simulink model "benchlink"  (R2024b)
settings: Solver=FixedStepDiscrete  StartTime=0.0  StopTime=0.005*16  RelTol=1e-3
model workspace (MAT data in the model file):
  socvcb = containers.Map
  socvcb.serialization.keys = {}
  socvcb.serialization.values = {}
  socvcb.serialization.uniformity = 0
  socvcb.serialization.keyType = 'double'
  socvcb.serialization.valueType = 'any'
values from neighbouring files (symbols this model uses):
  access = [32 0 4 36 32 0 4 36 32 0 4 36 ... (16 elements, 16x1)]    [all_variables.mat]
  qam_params =     [all_variables.mat]
undefined symbols (not defined in the file or in its folder): Add, j, QAM, rms, Shift
libraries: hdlsllib x53, simulink_need_slupdate x22, simulink x18, dspsigops x16, commdigbbndam3 x6, dsphdlmathfun2 x2, commchan3 x1, commrflib2 x1, dsphdlsigops2 x1, dspstat3 x1, dsphdlfiltering2 x1, simulink_extras x1
(part 1 of 5)
settings Model: ModifiedByFormat=The MathWorks Inc.  VariantFading=off  Creator=The MathWorks, Inc.  LastModifiedBy=The MathWorks Inc.
settings SolverCC: AlgebraicLoopSolver=TrustRegion  PositivePriorityOrder=on
settings DataIOCC: LimitDataPoints=on  SaveFormat=Array  SaveOutput=off  SaveTime=off  ReturnWorkspaceOutputs=off
settings OptimizationCC: BlockReduction=off  ConditionallyExecuteInputs=off  DefaultParameterBehavior=Inlined  EnhancedBackFolding=on  PassReuseOutputArgsAs=Individual arguments  MaxStackSize=64  OptimizeBlockOrder=speed  DifferentSizesBufferReuse=on  OptimizationCustomize=off  EfficientTunableParamExpr=on
settings DebuggingCC: AlgebraicLoopMsg=error  UnderspecifiedInitializationDetection=Classic  MergeDetectMultiDrivingBlocksExec=none  SolverPrmCheckMsg=warning  MultiTaskDSMMsg=warning  MultiTaskCondExecSysMsg=none  SingleTaskRateTransMsg=error  IntegerOverflowMsg=none  ParameterPrecisionLossMsg=none  ParameterTunabilityLossMsg=error  UnconnectedInputMsg=warning  UnconnectedOutputMsg=warning  UnconnectedLineMsg=warning  AllowSymbolicDim=off  StateNameClashWarn=warning  SFUnexpectedBacktrackingDiag=warning  SFNoUnconditionalDefaultTransitionDiag=warning  SFExecutionAtInitializationDiag=none  IntegerSaturationMsg=none  ArithmeticOperatorsInVariantConditions=warning
settings HardwareCC: ProdBitPerPointer=32  ProdBitPerSizeT=32  ProdBitPerPtrDiffT=32  ProdLargestAtomicFloat=None  ProdIntDivRoundTo=Undefined  ProdEndianess=Unspecified  ProdWordSize=32  ProdHWDeviceType=ASIC/FPGA->ASIC/FPGA  TargetBitPerLong=64  TargetBitPerPointer=64  TargetBitPerSizeT=64  TargetBitPerPtrDiffT=64  TargetLongLongMode=on  TargetIntDivRoundTo=Zero  TargetEndianess=LittleEndian  TargetWordSize=64  TargetHWDeviceType=Custom Processor->MATLAB Host Computer  ProdEqTarget=off
settings ModelReferenceCC: EnableRefExpFcnMdlSchedulingChecks=on  PropagateSignalLabelsOutOfModel=off
settings SFSimCC: SimUseLocalCustomCode=off  MATLABDynamicMemAlloc=off  CustomCodeUndefinedFunction=UseInterfaceOnly
settings RTWCC: Description=Embedded Coder  SystemTargetFile=ert.tlc  TemplateMakefile=ert_default_tmf  GenerateReport=on  RTWUseLocalCustomCode=off  Toolchain=Linaro AArch64 Linux v6.3.1  IncludeHyperlinkInReport=on  LaunchReport=on  GenerateTraceInfo=on  GenerateTraceReport=on  GenerateTraceReportSl=on  GenerateTraceReportSf=on  GenerateTraceReportEml=on  GPUComputeCapability=3.5  DLArmComputeVersion=19.05
settings CodeAppCC: ForceParamTrailComments=on  IgnoreCustomStorageClasses=off  OperatorAnnotations=on  SimulinkDataObjDesc=on  SFDataObjDesc=on  InsertBlockDesc=on
settings ERTTargetCC: InlinedParameterPlacement=Hierarchical  ERTCustomFileTemplate=example_file_process.tlc  DynamicArrayContainerType=coder::array
settings ConfigComp: CovMetricSettings=dw  CovSaveCumulativeToWorkspaceVar=on  CovSaveSingleToWorkspaceVar=on  CovExternalEMLEnable=off  CovSFcnEnable=off

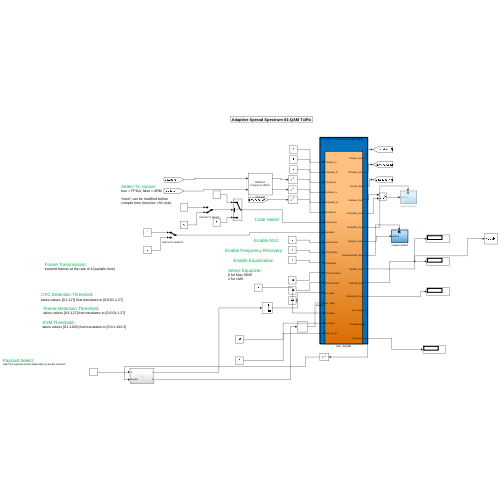
[thumbnail: Simulink's stored preview of the top-level diagram]
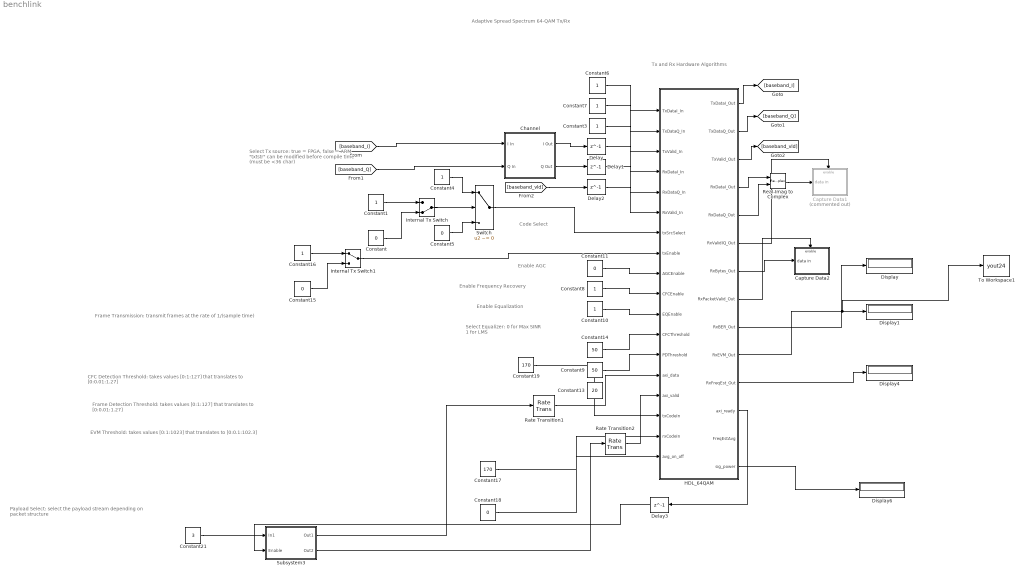
== system benchlink ==
  note: Adaptive Spread Spectrum 64-QAM Tx/Rx
  note: Tx and Rx Hardware Algorithms
  note: Select Tx source:
      | true = FPGA, false = ARM
      |
      | "txtstr" can be modified before
      | compile time (must be <36 char)
  note: Frame Transmission:
      | transmit frames at the rate of 1/(sample time)
  note: Code Select
  note: Enable Frequency Recovery
  note: Frame Detection Threshold:
      | takes values [0:1:127] that translates to [0:0.01:1.27]
  note: Enable Equalization
  note: Enable AGC
  note: Select Equalizer:
      | 0 for Max SINR
      | 1 for LMS
  note: EVM Threshold:
      | takes values [0:1:1023] that translates to [0:0.1:102.3]
  note: CFC Detection Threshold:
      | takes values [0:1:127] that translates to [0:0.01:1.27]
  note: Payload Select:
      | select the payload stream depending on packet structure
  Capture Data1 : Subsystem  Commented=on
  Capture Data2 : Subsystem
  Channel : Subsystem  mask{Poff=qam_params.phaseOffset, Foff=qam_params.frequencyOffset, EbNo=qam_params.EbNo, Chan_Gain=qam_params.channelGain, Chan_Delay=qam_params.channelDelay}
      mask prompts: Poff "Phase offset (deg)"; Foff "Frequency offset (Hz)"; EbNo "Eb/No"; Chan_Gain "Channel Gain"; Chan_Delay "Channel Delay"
      mask Display: disp('AWGN &\nFrequency Offset');
  Constant{,5,11,15,18} (5 alike) : Constant  Value=0  OutDataTypeStr=boolean  SampleTime=-1
  Constant{1,3..4,8,10,16} (6 alike) : Constant  OutDataTypeStr=boolean  SampleTime=-1
  Constant13 : Constant  Value=20  OutDataTypeStr=int16  SampleTime=-1
  Constant14 : Constant  Value=50  OutDataTypeStr=int16  SampleTime=-1
  Constant17 : Constant  Value=170  OutDataTypeStr=int16  SampleTime=-1
  Constant19 : Constant  Value=170  OutDataTypeStr=int16  SampleTime=-1
  Constant21 : Constant  Value=3  OutDataTypeStr=uint16  SampleTime=-1
  Constant6 : Constant  OutDataTypeStr=int16  SampleTime=-1
  Constant7 : Constant  OutDataTypeStr=int16  SampleTime=-1
  Constant9 : Constant  Value=50  OutDataTypeStr=int16  SampleTime=-1
  Delay{,1..3} (4 alike) : Delay  DelayLength=1
  Display{,1,4,6} (4 alike) : Display
  HDL_64QAM : Subsystem  TreatAsAtomicUnit=on
  Internal Tx Switch : ManualSwitch  CurrentSetting=0
  Internal Tx Switch1 : ManualSwitch
  Rate Transition1 : RateTransition  OutPortSampleTime=1/qam_params.sampleRate
  Rate Transition2 : RateTransition  OutPortSampleTime=1/qam_params.sampleRate
  Real-Imag to Complex : RealImagToComplex
  Subsystem3 : Subsystem
  Switch : Switch  Criteria=u2 ~= 0  SaturateOnIntegerOverflow=off  InputSameDT=off
  To Workspace1 : ToWorkspace  VariableName=yout24  SampleTime=-1
      settings: Save2DSignal=2-D array (concatenate along first dimension)
  wires:
  Internal Tx Switch/1 -> Switch/2
  [baseband_vld] -> Delay2/1
  Constant5/1 -> Switch/3
  Constant/1 -> Internal Tx Switch/2
  Constant4/1 -> Switch/1
  Constant1/1 -> Internal Tx Switch/1
  HDL_64QAM/1(TxDataI_Out) -> [baseband_I]
  HDL_64QAM/2(TxDataQ_Out) -> [baseband_Q]
  HDL_64QAM/3(TxValid_Out) -> [baseband_vld]
  Delay/1 -> HDL_64QAM/4(RxDataI_In)
  Delay2/1 -> HDL_64QAM/6(RxValid_In)
  Switch/1 -> HDL_64QAM/7(txSrcSelect)
  Delay1/1 -> HDL_64QAM/5(RxDataQ_In)
  Constant6/1 -> HDL_64QAM/1(TxDataI_In)
  Constant7/1 -> HDL_64QAM/2(TxDataQ_In)
  Constant3/1 -> HDL_64QAM/3(TxValid_In)
  Real-Imag to Complex/1 -> Capture Data1/1(data in)
  HDL_64QAM/6(RxValidIQ_Out) -> Capture Data1/Enable
  HDL_64QAM/5(RxDataQ_Out) -> Real-Imag to Complex/2
  HDL_64QAM/4(RxDataI_Out) -> Real-Imag to Complex/1
  Constant8/1 -> HDL_64QAM/10(CFCEnable)
  Constant9/1 -> HDL_64QAM/13(PDThreshold)
  Constant10/1 -> HDL_64QAM/11(EQEnable)
  Constant11/1 -> HDL_64QAM/9(AGCEnable)
  HDL_64QAM/10(RxEVM_Out) -> To Workspace1/1, Display1/1
  HDL_64QAM/9(RxBER_Out) -> Display/1
  HDL_64QAM/11(RxFreqEst_Out) -> Display4/1
  Constant14/1 -> HDL_64QAM/12(CFCThreshold)
  HDL_64QAM/12(axi_ready) -> Delay3/1
  HDL_64QAM/7(RxBytes_Out) -> Capture Data2/1(data in)
  HDL_64QAM/8(RxPacketValid_Out) -> Capture Data2/Enable
  Internal Tx Switch1/1 -> HDL_64QAM/8(txEnable)
  Constant15/1 -> Internal Tx Switch1/2
  Constant16/1 -> Internal Tx Switch1/1
  Rate Transition1/1 -> HDL_64QAM/14(axi_data)
  Rate Transition2/1 -> HDL_64QAM/15(axi_valid)
  Constant17/1 -> HDL_64QAM/17(rxCodeIn)
  Constant19/1 -> HDL_64QAM/16(txCodeIn)
  [baseband_I] -> Channel/1(I In)
  [baseband_Q] -> Channel/2(Q In)
  Constant18/1 -> HDL_64QAM/18(avg_on_off)
  HDL_64QAM/14(sig_power) -> Display6/1
  Constant21/1 -> Subsystem3/1(In1)
  Delay3/1 -> Subsystem3/2(Enable)
  Subsystem3/1(Out1) -> Rate Transition1/1
  Subsystem3/2(Out2) -> Rate Transition2/1
  Channel/1(I Out) -> Delay/1
  Channel/2(Q Out) -> Delay1/1

== system benchlink/Capture Data1 ==
  data in : Inport
  Enable : EnablePort
  Constellation Diagram : ConstellationDiagram  WindowPosition=[67.000000,1.000000,612.000000,254.000000,]  ScopeFrameLocation=window  SymbolsToDisplaySource=Property  SymbolsToDisplay=2048  ReferenceConstellation=64-QAM  DefaultConfigurationName=comm.scopes.ConstellationDiagramBlockCfg
  wires:
  data in/1 -> Constellation Diagram/1

== system benchlink/Capture Data2 ==
  data in : Inport
  Enable : EnablePort
  To Workspace : ToWorkspace  VariableName=outout  SampleTime=-1
      settings: Save2DSignal=2-D array (concatenate along first dimension)
  wires:
  data in/1 -> To Workspace/1

== system benchlink/Channel ==
  I In : Inport
  Q In : Inport  Port=2
  AWGN Channel2 : commchan3/AWGN Channel  LegacyMode=on  NoiseMethod="Signal to noise ratio  (SNR)"  noiseMode="Signal to noise ratio  (Eb/No)"  EbNo=EbNo  EsNo=15  SNR=15  BitsPerSymbol=6  SignalPower=0.21  SamplesPerSymbol=1  SymbolPeriod=1/qam_params.sampleRate  VarianceSource=Parameter  Variance=1  RandomStream=Global stream  Seed=67  SimulateUsing=Code generation
  Complex to Real-Imag : ComplexToRealImag
  Constant : Constant  Value=Chan_Delay  SampleTime=1/qam_params.sampleRate
  Data Type Conversion1 : DataTypeConversion  OutDataTypeStr=fixdt(1,16,15)  SaturateOnIntegerOverflow=off  RndMeth=Floor
  Data Type Conversion4 : DataTypeConversion  OutDataTypeStr=double  SaturateOnIntegerOverflow=off  RndMeth=Floor
  Gain : Gain  Gain=Chan_Gain
  Phase/ Frequency Offset1 : commrflib2/Phase// Frequency Offset  phaseOffset=Poff  freqPort=off  freqOffset=Foff
  Real-Imag to Complex : RealImagToComplex
  Variable Fractional Delay : dspsigops/Variable Fractional Delay  mode=OBSOLETE  modeActive=Linear  L=4  FarrowL=4  R=10  alpha=1  dmax=56*4  ic=0  noDFT=off  fallbackFIR=Clip to the minimum value necessary for centered kernel  fallbackFarrow=Clip to the minimum value necessary for centered kernel  roundingMode=Zero  overflowMode=off
  I Out : Outport  VectorParamsAs1DForOutWhenUnconnected=off
  Q Out : Outport  Port=2  VectorParamsAs1DForOutWhenUnconnected=off
  wires:
  AWGN Channel2/1 -> Gain/1
  Data Type Conversion4/1 -> Phase/ Frequency Offset1/1
  Phase/ Frequency Offset1/1 -> Variable Fractional Delay/1
  Variable Fractional Delay/1 -> AWGN Channel2/1
  Constant/1 -> Variable Fractional Delay/2
  Gain/1 -> Data Type Conversion1/1
  Real-Imag to Complex/1 -> Data Type Conversion4/1
  I In/1 -> Real-Imag to Complex/1
  Q In/1 -> Real-Imag to Complex/2
  Data Type Conversion1/1 -> Complex to Real-Imag/1
  Complex to Real-Imag/1 -> I Out/1
  Complex to Real-Imag/2 -> Q Out/1

== system benchlink/HDL_64QAM ==
  TxDataI_In : Inport
  TxDataQ_In : Inport  Port=2
  TxValid_In : Inport  Port=3
  RxDataI_In : Inport  Port=4
  RxDataQ_In : Inport  Port=5
  RxValid_In : Inport  Port=6
  txSrcSelect : Inport  Port=7
  txEnable : Inport  Port=8
  AGCEnable : Inport  Port=9
  CFCEnable : Inport  Port=10
  EQEnable : Inport  Port=11
  CFCThreshold : Inport  Port=12
  PDThreshold : Inport  Port=13
  axi_data : Inport  Port=14
  axi_valid : Inport  Port=15  OutDataTypeStr=boolean
  txCodeIn : Inport  Port=16
  rxCodeIn : Inport  Port=17
  avg_on_off : Inport  Port=18
  Constant20 : Constant  Value=8  OutDataTypeStr=uint16  SampleTime=-1
  Constant22 : Constant  Value=4  OutDataTypeStr=uint16  SampleTime=-1
  HDLRxIPCore : Subsystem  TreatAsAtomicUnit=on
  HDLTxIPCore : Subsystem  TreatAsAtomicUnit=on
  TxDataI_Out : Outport  VectorParamsAs1DForOutWhenUnconnected=off
  TxDataQ_Out : Outport  Port=2  VectorParamsAs1DForOutWhenUnconnected=off
  TxValid_Out : Outport  Port=3  VectorParamsAs1DForOutWhenUnconnected=off
  RxDataI_Out : Outport  Port=4  VectorParamsAs1DForOutWhenUnconnected=off
  RxDataQ_Out : Outport  Port=5  VectorParamsAs1DForOutWhenUnconnected=off
  RxValidIQ_Out : Outport  Port=6  VectorParamsAs1DForOutWhenUnconnected=off
  RxBytes_Out : Outport  Port=7  VectorParamsAs1DForOutWhenUnconnected=off
  RxPacketValid_Out : Outport  Port=8  VectorParamsAs1DForOutWhenUnconnected=off
  RxBER_Out : Outport  Port=9  VectorParamsAs1DForOutWhenUnconnected=off
  RxEVM_Out : Outport  Port=10  VectorParamsAs1DForOutWhenUnconnected=off
  RxFreqEst_Out : Outport  Port=11  VectorParamsAs1DForOutWhenUnconnected=off
  axi_ready : Outport  Port=12
  FreqEstAvg : Outport  Port=13  VectorParamsAs1DForOutWhenUnconnected=off
  sig_power : Outport  Port=14  PortDimensions=1  VectorParamsAs1DForOutWhenUnconnected=off
  wires:
  HDLRxIPCore/10(sig_power) -> sig_power/1
  HDLRxIPCore/8(FreqEst_Out) -> RxFreqEst_Out/1
  HDLRxIPCore/7(EVM_Out) -> RxEVM_Out/1
  HDLRxIPCore/6(BER_Out) -> RxBER_Out/1
  rxCodeIn/1 -> HDLRxIPCore/4(codeSequence)
  RxDataQ_In/1 -> HDLRxIPCore/2(Imag_In)
  HDLRxIPCore/9(FreqEstAvg) -> FreqEstAvg/1
  HDLTxIPCore/2(Imag_Out) -> TxDataQ_Out/1
  TxValid_In/1 -> HDLTxIPCore/3(Valid_In)
  Constant22/1 -> HDLRxIPCore/11(fineCorrections), HDLTxIPCore/9(access_per_burst)
  HDLRxIPCore/5(PacketValid_Out) -> RxPacketValid_Out/1
  txEnable/1 -> HDLTxIPCore/6(txEnable)
  Constant20/1 -> HDLTxIPCore/10(packetsPerBurst), HDLRxIPCore/12(packetsPerBurst)
  txCodeIn/1 -> HDLTxIPCore/5(codeSequence)
  RxValid_In/1 -> HDLRxIPCore/3(Valid_In)
  CFCEnable/1 -> HDLRxIPCore/6(CFCEnable)
  HDLRxIPCore/2(Imag_Out) -> RxDataQ_Out/1
  axi_data/1 -> HDLTxIPCore/7(axi_data)
  TxDataQ_In/1 -> HDLTxIPCore/2(Imag_In)
  RxDataI_In/1 -> HDLRxIPCore/1(Real_In)
  axi_valid/1 -> HDLTxIPCore/8(axi_valid)
  HDLTxIPCore/1(Real_Out) -> TxDataI_Out/1
  txSrcSelect/1 -> HDLTxIPCore/4(txSrcSelect)
  TxDataI_In/1 -> HDLTxIPCore/1(Real_In)
  EQEnable/1 -> HDLRxIPCore/7(EQEnable)
  CFCThreshold/1 -> HDLRxIPCore/8(CFCThreshold)
  PDThreshold/1 -> HDLRxIPCore/9(PDThreshold)
  AGCEnable/1 -> HDLRxIPCore/5(AGCEnable)
  HDLRxIPCore/3(Valid_IQ) -> RxValidIQ_Out/1
  avg_on_off/1 -> HDLRxIPCore/10(avg_on_off)
  HDLRxIPCore/1(Real_Out) -> RxDataI_Out/1
  HDLTxIPCore/3(Valid_Out) -> TxValid_Out/1
  HDLTxIPCore/4(axi_ready) -> axi_ready/1
  HDLRxIPCore/4(Bytes_Out) -> RxBytes_Out/1

== system benchlink/Subsystem3 ==
  In1 : Inport
  Enable : Inport  Port=2
  AXI_Write_x_in_DTC{,1..3} (4 alike) : DataTypeConversion  OutDataTypeStr=uint32  ConvertRealWorld=Stored Integer (SI)  SaturateOnIntegerOverflow=off  RndMeth=Floor
  From Workspace : FromWorkspace  VariableName=streamdata  OutDataTypeStr=double  SampleTime=1/qam_params.sampleRate*240  Interpolate=off  OutputAfterFinalValue=Cyclic repetition
  From Workspace1 : FromWorkspace  VariableName=streamdata_224  OutDataTypeStr=double  SampleTime=1/qam_params.sampleRate*224  Interpolate=off  OutputAfterFinalValue=Cyclic repetition
  From Workspace2 : FromWorkspace  VariableName=streamdata_192  OutDataTypeStr=double  SampleTime=1/qam_params.sampleRate*192  Interpolate=off  OutputAfterFinalValue=Cyclic repetition
  From Workspace3 : FromWorkspace  VariableName=streamdata_128  OutDataTypeStr=double  SampleTime=1/qam_params.sampleRate*128  Interpolate=off  OutputAfterFinalValue=Cyclic repetition
  Multiport Switch : MultiPortSwitch  Inputs=4  SaturateOnIntegerOverflow=off  InputSameDT=off
  Multiport Switch1 : MultiPortSwitch  Inputs=4  SaturateOnIntegerOverflow=off  InputSameDT=off
  Subsystem : Subsystem
  Subsystem1 : Subsystem
  Subsystem2 : Subsystem
  Subsystem3 : Subsystem
  Out1 : Outport
  Out2 : Outport  Port=2
  wires:
  AXI_Write_x_in_DTC/1 -> Subsystem/1(P)
  Subsystem/2(ValidOut) -> Multiport Switch1/2
  Subsystem2/2(ValidOut) -> Multiport Switch1/4
  From Workspace2/1 -> AXI_Write_x_in_DTC2/1
  Subsystem1/1(S) -> Multiport Switch/3
  Subsystem1/2(ValidOut) -> Multiport Switch1/3
  Multiport Switch1/1 -> Out2/1
  Subsystem2/1(S) -> Multiport Switch/4
  Enable/1 -> Subsystem3/Enable, Subsystem2/Enable, Subsystem1/Enable, Subsystem/Enable
  In1/1 -> Multiport Switch1/1, Multiport Switch/1
  Multiport Switch/1 -> Out1/1
  AXI_Write_x_in_DTC1/1 -> Subsystem1/1(P)
  From Workspace/1 -> AXI_Write_x_in_DTC/1
  Subsystem/1(S) -> Multiport Switch/2
  AXI_Write_x_in_DTC2/1 -> Subsystem2/1(P)
  From Workspace1/1 -> AXI_Write_x_in_DTC1/1
  From Workspace3/1 -> AXI_Write_x_in_DTC3/1
  AXI_Write_x_in_DTC3/1 -> Subsystem3/1(P)
  Subsystem3/1(S) -> Multiport Switch/5
  Subsystem3/2(ValidOut) -> Multiport Switch1/5

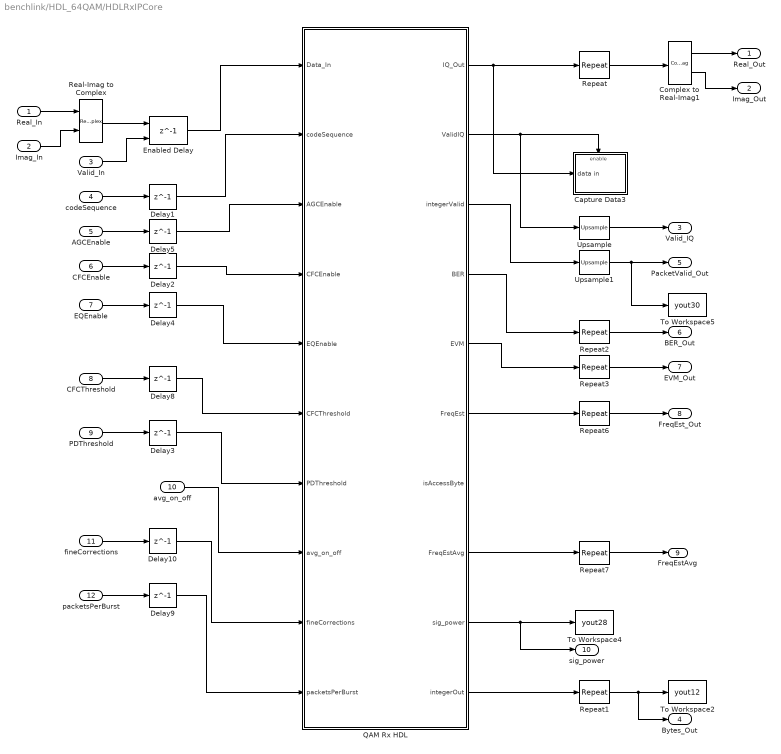
== system benchlink/HDL_64QAM/HDLRxIPCore ==
  Real_In : Inport
  Imag_In : Inport  Port=2
  Valid_In : Inport  Port=3
  codeSequence : Inport  Port=4
  AGCEnable : Inport  Port=5
  CFCEnable : Inport  Port=6
  EQEnable : Inport  Port=7
  CFCThreshold : Inport  Port=8
  PDThreshold : Inport  Port=9
  avg_on_off : Inport  Port=10
  fineCorrections : Inport  Port=11
  packetsPerBurst : Inport  Port=12
  Capture Data3 : Subsystem
  Complex to Real-Imag1 : ComplexToRealImag
  Delay{1..5,8..10} (8 alike) : Delay  DelayLength=1
  Enabled Delay : Delay  DelayLength=1  ShowEnablePort=on
      settings: InputPortMap=u0,e6
  QAM Rx HDL : Subsystem
  Real-Imag to Complex : RealImagToComplex
  Repeat{,1..3,6..7} (6 alike) : dspsigops/Repeat  FactorSource=Dialog parameter  N=qam_params.Upsampling  Nmax=16  InputProcessing=Columns as channels (frame based)  RateOptions=Allow multirate processing  ic=0  mode=Unused parameter value
  To Workspace2 : ToWorkspace  VariableName=yout12  SampleTime=-1
      settings: Save2DSignal=2-D array (concatenate along first dimension)
  To Workspace4 : ToWorkspace  VariableName=yout28  SampleTime=-1
      settings: Save2DSignal=2-D array (concatenate along first dimension)
  To Workspace5 : ToWorkspace  VariableName=yout30  SampleTime=-1
      settings: Save2DSignal=2-D array (concatenate along first dimension)
  Upsample : dspsigops/Upsample  FactorSource=Dialog parameter  N=qam_params.Upsampling  Nmax=16  phase=0  InputProcessing=Columns as channels (frame based)  RateOptions=Allow multirate processing  ic=0  mode=Unused parameter value
  Upsample1 : dspsigops/Upsample  FactorSource=Dialog parameter  N=qam_params.Upsampling  Nmax=16  phase=0  InputProcessing=Columns as channels (frame based)  RateOptions=Allow multirate processing  ic=0  mode=Unused parameter value
  Real_Out : Outport  VectorParamsAs1DForOutWhenUnconnected=off
  Imag_Out : Outport  Port=2  VectorParamsAs1DForOutWhenUnconnected=off
  Valid_IQ : Outport  Port=3  VectorParamsAs1DForOutWhenUnconnected=off
  Bytes_Out : Outport  Port=4  VectorParamsAs1DForOutWhenUnconnected=off
  PacketValid_Out : Outport  Port=5  VectorParamsAs1DForOutWhenUnconnected=off
  BER_Out : Outport  Port=6  VectorParamsAs1DForOutWhenUnconnected=off
  EVM_Out : Outport  Port=7  VectorParamsAs1DForOutWhenUnconnected=off
  FreqEst_Out : Outport  Port=8  VectorParamsAs1DForOutWhenUnconnected=off
  FreqEstAvg : Outport  Port=9  VectorParamsAs1DForOutWhenUnconnected=off
  sig_power : Outport  Port=10  PortDimensions=1  VectorParamsAs1DForOutWhenUnconnected=off
  wires:
  Complex to Real-Imag1/2 -> Imag_Out/1
  Repeat6/1 -> FreqEst_Out/1
  Repeat3/1 -> EVM_Out/1
  Repeat2/1 -> BER_Out/1
  Repeat/1 -> Complex to Real-Imag1/1
  QAM Rx HDL/10(integerOut) -> Repeat1/1
  QAM Rx HDL/8(FreqEstAvg) -> Repeat7/1
  Complex to Real-Imag1/1 -> Real_Out/1
  QAM Rx HDL/5(EVM) -> Repeat3/1
  QAM Rx HDL/4(BER) -> Repeat2/1
  QAM Rx HDL/9(sig_power) -> To Workspace4/1, sig_power/1
  QAM Rx HDL/3(integerValid) -> Upsample1/1
  Repeat1/1 -> Bytes_Out/1, To Workspace2/1
  Enabled Delay/1 -> QAM Rx HDL/1(Data_In)
  CFCThreshold/1 -> Delay8/1
  PDThreshold/1 -> Delay3/1
  EQEnable/1 -> Delay4/1
  Repeat7/1 -> FreqEstAvg/1
  QAM Rx HDL/1(IQ_Out) -> Repeat/1, Capture Data3/1(data in)
  fineCorrections/1 -> Delay10/1
  CFCEnable/1 -> Delay2/1
  avg_on_off/1 -> QAM Rx HDL/8(avg_on_off)
  Upsample/1 -> Valid_IQ/1
  QAM Rx HDL/2(ValidIQ) -> Upsample/1, Capture Data3/Enable
  AGCEnable/1 -> Delay5/1
  Valid_In/1 -> Enabled Delay/2
  codeSequence/1 -> Delay1/1
  Upsample1/1 -> PacketValid_Out/1, To Workspace5/1
  Imag_In/1 -> Real-Imag to Complex/2
  Real_In/1 -> Real-Imag to Complex/1
  Delay8/1 -> QAM Rx HDL/6(CFCThreshold)
  Real-Imag to Complex/1 -> Enabled Delay/1
  Delay1/1 -> QAM Rx HDL/2(codeSequence)
  Delay5/1 -> QAM Rx HDL/3(AGCEnable)
  Delay2/1 -> QAM Rx HDL/4(CFCEnable)
  packetsPerBurst/1 -> Delay9/1
  Delay4/1 -> QAM Rx HDL/5(EQEnable)
  Delay10/1 -> QAM Rx HDL/9(fineCorrections)
  Delay9/1 -> QAM Rx HDL/10(packetsPerBurst)
  Delay3/1 -> QAM Rx HDL/7(PDThreshold)
  QAM Rx HDL/6(FreqEst) -> Repeat6/1

== system benchlink/HDL_64QAM/HDLTxIPCore ==
  Real_In : Inport
  Imag_In : Inport  Port=2
  Valid_In : Inport  Port=3
  txSrcSelect : Inport  Port=4
  codeSequence : Inport  Port=5
  txEnable : Inport  Port=6
  axi_data : Inport  Port=7
  axi_valid : Inport  Port=8  OutDataTypeStr=boolean
  access_per_burst : Inport  Port=9
  packetsPerBurst : Inport  Port=10
  Complex to Real-Imag1 : ComplexToRealImag
  Delay : Delay  DelayLength=1
  Delay1 : Delay  DelayLength=1
  Delay2 : Delay  DelayLength=1  InitialCondition=0
  Enabled Delay : Delay  DelayLength=1  ShowEnablePort=on
      settings: InputPortMap=u0,e6
  QAMTxHDL : Subsystem
  Real-Imag to Complex : RealImagToComplex
  Real_Out : Outport  VectorParamsAs1DForOutWhenUnconnected=off
  Imag_Out : Outport  Port=2  VectorParamsAs1DForOutWhenUnconnected=off
  Valid_Out : Outport  Port=3  VectorParamsAs1DForOutWhenUnconnected=off
  axi_ready : Outport  Port=4
  wires:
  Complex to Real-Imag1/1 -> Real_Out/1
  Complex to Real-Imag1/2 -> Imag_Out/1
  QAMTxHDL/1(Data_Out) -> Complex to Real-Imag1/1
  QAMTxHDL/2(Valid Out) -> Valid_Out/1
  Real-Imag to Complex/1 -> Enabled Delay/1
  Valid_In/1 -> Enabled Delay/2, QAMTxHDL/7(validInCh1)
  Real_In/1 -> Real-Imag to Complex/1
  Imag_In/1 -> Real-Imag to Complex/2
  txSrcSelect/1 -> Delay/1
  codeSequence/1 -> Delay1/1
  Delay1/1 -> QAMTxHDL/1(codeSequence)
  txEnable/1 -> QAMTxHDL/2(txEnable)
  Delay/1 -> QAMTxHDL/3(txSrcSelect)
  Enabled Delay/1 -> QAMTxHDL/6(dataInCh1)
  axi_data/1 -> QAMTxHDL/4(data_in)
  axi_valid/1 -> QAMTxHDL/5(valid_in)
  QAMTxHDL/3(axi_ready) -> axi_ready/1
  access_per_burst/1 -> QAMTxHDL/8(access_per_burst)
  packetsPerBurst/1 -> Delay2/1
  Delay2/1 -> QAMTxHDL/9(packetsPerBurst)

== system benchlink/Subsystem3/Subsystem ==
  P : Inport
  Enable : EnablePort
  Serializer1D : hdlsllib/HDL Operations/Serializer1D  Ratio=240  IdleCycles=0  validIn=off  startOut=off  validOut=on  inputDataDimensions=-1  inputSampleTime=-1  inputSignalType=auto
  S : Outport
  ValidOut : Outport  Port=2
  wires:
  Serializer1D/2 -> ValidOut/1
  Serializer1D/1 -> S/1
  P/1 -> Serializer1D/1

== system benchlink/Subsystem3/Subsystem1 ==
  P : Inport
  Enable : EnablePort
  Serializer1D : hdlsllib/HDL Operations/Serializer1D  Ratio=224  IdleCycles=0  validIn=off  startOut=off  validOut=on  inputDataDimensions=-1  inputSampleTime=-1  inputSignalType=auto
  S : Outport
  ValidOut : Outport  Port=2
  wires:
  Serializer1D/2 -> ValidOut/1
  Serializer1D/1 -> S/1
  P/1 -> Serializer1D/1

== system benchlink/Subsystem3/Subsystem2 ==
  P : Inport
  Enable : EnablePort
  Serializer1D : hdlsllib/HDL Operations/Serializer1D  Ratio=192  IdleCycles=0  validIn=off  startOut=off  validOut=on  inputDataDimensions=-1  inputSampleTime=-1  inputSignalType=auto
  S : Outport
  ValidOut : Outport  Port=2
  wires:
  Serializer1D/2 -> ValidOut/1
  Serializer1D/1 -> S/1
  P/1 -> Serializer1D/1

== system benchlink/Subsystem3/Subsystem3 ==
  P : Inport
  Enable : EnablePort
  Serializer1D : hdlsllib/HDL Operations/Serializer1D  Ratio=128  IdleCycles=0  validIn=off  startOut=off  validOut=on  inputDataDimensions=-1  inputSampleTime=-1  inputSignalType=auto
  S : Outport
  ValidOut : Outport  Port=2
  wires:
  Serializer1D/2 -> ValidOut/1
  Serializer1D/1 -> S/1
  P/1 -> Serializer1D/1

== system benchlink/HDL_64QAM/HDLRxIPCore/Capture Data3 ==
  data in : Inport
  Enable : EnablePort
  Constellation Diagram : ConstellationDiagram  WindowPosition=[67.000000,1.000000,3374.000000,1371.000000,]  ScopeFrameLocation=window  SymbolsToDisplaySource=Property  SymbolsToDisplay=2048  ReferenceConstellation=64-QAM  DefaultConfigurationName=comm.scopes.ConstellationDiagramBlockCfg
  wires:
  data in/1 -> Constellation Diagram/1

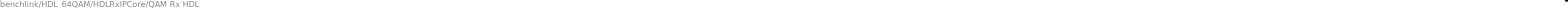
== system benchlink/HDL_64QAM/HDLRxIPCore/QAM Rx HDL ==
  note: Enabled AGC1: use gain = 0.01 for both sim/impl
      | Enabled AGC3: use gain = 0.0001/0.001 for sim/impl
  Data_In : Inport
  codeSequence : Inport  Port=2
  AGCEnable : Inport  Port=3
  CFCEnable : Inport  Port=4
  EQEnable : Inport  Port=5
  CFCThreshold : Inport  Port=6
  PDThreshold : Inport  Port=7
  avg_on_off : Inport  Port=8
  fineCorrections : Inport  Port=9
  packetsPerBurst : Inport  Port=10
  AGC Enable : Subsystem
  CFC Enable : Subsystem
  CFC Threshold : Subsystem
  Complex to Real-Imag4 : ComplexToRealImag
  Complex to Real-Imag6 : ComplexToRealImag
  Constant6 : Constant  OutDataTypeStr=boolean  SampleTime=-1
  DA CFC_Avg : Subsystem
  Data Type Conversion3 : DataTypeConversion  OutDataTypeStr=fixdt(0,16,9)
  Delay{1..3,5..6,8..9,12,14,16..17,20,22..23,26..27,31..33,45} (20 alike) : Delay  DelayLength=1  InitialCondition=0
  EB Downsampler by 6 : Subsystem  mask{M=128}
      mask prompts: M "FIR Length"
  EB Downsampler by 6_Old2 : Subsystem  Commented=on  mask{M=128}
      mask prompts: M "FIR Length"
  EB Downsampler by 6_old : Subsystem  Commented=on  mask{M=128}
      mask prompts: M "FIR Length"
  EQ Enable : Subsystem
  Enabled AGC1 : Subsystem  Commented=on  mask{AGC_Ref=.23, AGC_Gain=0.01}
      mask prompts: AGC_Ref "Target Amplitude"; AGC_Gain "AGC Loop Gain"
  Enabled AGC2 : Subsystem  mask{AGC_Ref=.23, AGC_Gain=0.001}
      mask prompts: AGC_Ref "Target Amplitude"; AGC_Gain "AGC Loop Gain"
  MF Filtering and Despreading : Subsystem  mask{AccessSym=qam_params.longTrainingChips.', N=qam_params.longTrainingChipLength}
      mask prompts: AccessSym "Access code symbols"; N "Length of access code symbols"
  PD Threshold : Subsystem
  Payload Delimiter : Subsystem  mask{PreAmb=qam_params.golaySymbols.', threshold=0.6}
      mask prompts: PreAmb "Preamble symbols"
  SRRC : dsphdlfiltering2/Discrete FIR Filter  NumeratorSource=Property  Numerator=qam_params.ReceiverFilterCoefficients  NumeratorPrototype=[ 0.5, 0.5 ]  FilterStructure=Direct form transposed  SerializationOption=Minimum number of cycles between valid input samples  NumCycles=2  NumberOfMultipliers=2  SimulateUsing=Code generation  roundingMode=Floor  overflowMode=on  CoefficientsDataTypeStr=Inherit: Same word length as input  OutputDataTypeStr=fixdt(1,16,15)  ResetInputPort=off  HDLGlobalReset=off  CoeffMultiplier=Multiplier  UseMultForPow2Coeff=on
  Scope : Scope
  Terminator{5,8..9,12..14} (6 alike) : Terminator
  burstControl : MATLAB Function  TreatAsAtomicUnit=on
  IQ_Out : Outport  VectorParamsAs1DForOutWhenUnconnected=off
  ValidIQ : Outport  Port=2  VectorParamsAs1DForOutWhenUnconnected=off
  integerValid : Outport  Port=3  VectorParamsAs1DForOutWhenUnconnected=off
  BER : Outport  Port=4  VectorParamsAs1DForOutWhenUnconnected=off
  EVM : Outport  Port=5  VectorParamsAs1DForOutWhenUnconnected=off
  FreqEst : Outport  Port=6  VectorParamsAs1DForOutWhenUnconnected=off
  isAccessByte : Outport  Port=7  InitialOutput=0  VectorParamsAs1DForOutWhenUnconnected=off
  FreqEstAvg : Outport  Port=8  VectorParamsAs1DForOutWhenUnconnected=off
  sig_power : Outport  Port=9  PortDimensions=1  VectorParamsAs1DForOutWhenUnconnected=off
  integerOut : Outport  Port=10  VectorParamsAs1DForOutWhenUnconnected=off
  wires:
  Data Type Conversion3/1 -> BER/1  "BEROut"
  Delay33/1 -> EVM/1, [symEVM]  "EVMOut"
  Delay32/1 -> [BER], Data Type Conversion3/1
  Delay31/1 -> [ChCoeff]
  fineCorrections/1 -> Payload Delimiter/3(fineCorrections)
  burstControl/1(switchControl) -> Payload Delimiter/4(switchControl), MF Filtering and Despreading/6(switchControl), DA CFC_Avg/5(switchControl)
  Delay27/1 -> DA CFC_Avg/2(CFCEnable)  "CFCEnIn"
  CFC Threshold/1(Threshold) -> DA CFC_Avg/3(Threshold)
  packetsPerBurst/1 -> burstControl/1(packetsPerBurst)
  Delay8/1 -> DA CFC_Avg/1(dataIn)
  SRRC/1 -> Delay12/1
  Enabled AGC2/3(sig_power) -> sig_power/1
  Enabled AGC2/1(gain) -> Terminator5/1  "AGCGain"
  Delay5/1 -> CFC Enable/1(CFCEnable)
  DA CFC_Avg/2(FreqEst) -> Scope/1, FreqEst/1  "FreqEst"
  Delay2/1 -> Enabled AGC2/1(x), Complex to Real-Imag6/1
  CFCEnable/1 -> Delay5/1
  avg_on_off/1 -> DA CFC_Avg/4(avg_on_off)
  EQEnable/1 -> EQ Enable/1(EQEnable)
  CFC Enable/1(Out) -> Delay27/1
  Constant6/1 -> SRRC/2
  DA CFC_Avg/1(dataOut) -> Delay45/1
  CFCThreshold/1 -> CFC Threshold/1(CFCThreshold)
  Data_In/1 -> Delay2/1
  Delay12/1 -> EB Downsampler by 6/1(dataIn)
  Delay23/1 -> integerOut/1  "Integer"
  AGCEnable/1 -> AGC Enable/1(AGCEnable)
  Delay26/1 -> SRRC/1
  Complex to Real-Imag6/2 -> Terminator13/1  "AGCIn_Im"
  AGC Enable/1(Out) -> Enabled AGC2/2(AGCEnable)
  Complex to Real-Imag6/1 -> Terminator12/1  "AGCIn_Re"
  EB Downsampler by 6/1(dataOut) -> Delay8/1
  MF Filtering and Despreading/8(isAccessByte) -> Delay9/1
  Enabled AGC2/2(y) -> Delay26/1
  DA CFC_Avg/3(FreqEstAvg) -> FreqEstAvg/1
  PDThreshold/1 -> PD Threshold/1(PDThreshold)
  Complex to Real-Imag4/2 -> Terminator9/1  "PDOut_Im"
  Complex to Real-Imag4/1 -> Terminator8/1  "PDOut_Re"
  Delay3/1 -> MF Filtering and Despreading/5(EQEnable)  "EQEnable_In"
  Payload Delimiter/1(valid) -> Delay14/1
  Payload Delimiter/2(output) -> Delay16/1
  Payload Delimiter/3(isAccess) -> Delay17/1
  codeSequence/1 -> Delay6/1
  EQ Enable/1(Out) -> Delay3/1
  Delay9/1 -> isAccessByte/1
  burstControl/2(packetSymLength) -> Payload Delimiter/5(packetSymLength)
  SRRC/2 -> Terminator14/1
  Delay14/1 -> MF Filtering and Despreading/1(vaild_in)  "PDValid_Out"
  Delay16/1 -> MF Filtering and Despreading/2(input), Complex to Real-Imag4/1
  Delay17/1 -> MF Filtering and Despreading/3(isAccess)  "PDisAccess_Out"
  Delay6/1 -> MF Filtering and Despreading/4(codeSequence)  "EQcodeSeq_In"
  MF Filtering and Despreading/1(valid) -> Delay20/1
  MF Filtering and Despreading/5(ChCoeffOut) -> Delay31/1
  PD Threshold/1(Out) -> Payload Delimiter/2(Threshold)
  MF Filtering and Despreading/2(SymOut) -> Delay1/1
  MF Filtering and Despreading/4(IntOut) -> Delay23/1
  MF Filtering and Despreading/6(BEROut) -> Delay32/1
  MF Filtering and Despreading/3(validInt) -> Delay22/1
  MF Filtering and Despreading/7(SymEVMOut) -> Delay33/1
  Delay20/1 -> ValidIQ/1
  Delay1/1 -> IQ_Out/1
  Delay45/1 -> Payload Delimiter/1(Input)
  Delay22/1 -> integerValid/1

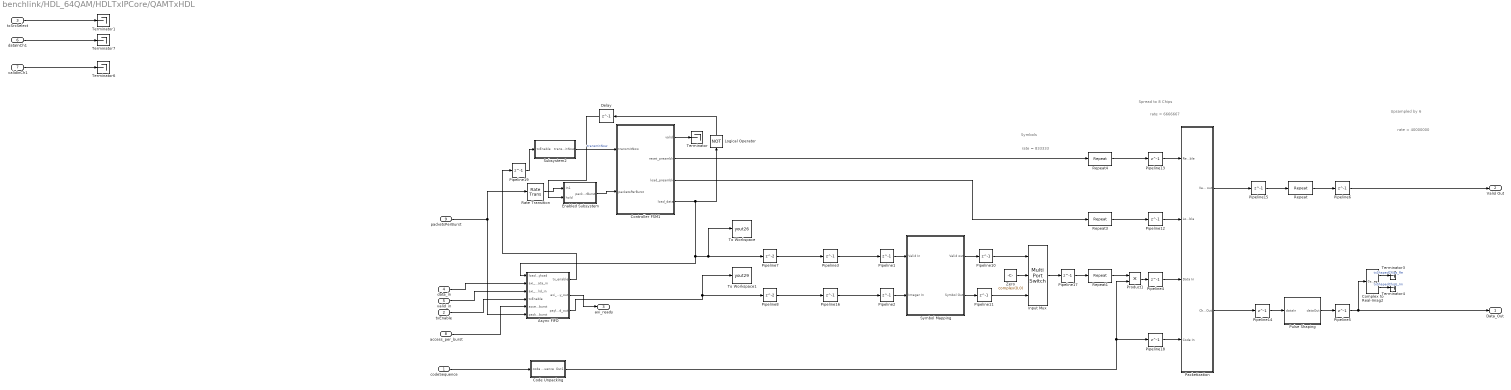
== system benchlink/HDL_64QAM/HDLTxIPCore/QAMTxHDL ==
  note: rate = 833333
  note: Spread to 8 Chips
  note: Symbols
  note: Upsampled by 6
  note: rate = 6666667
  note: rate = 40000000
  codeSequence : Inport
  txEnable : Inport  Port=2
  txSrcSelect : Inport  Port=3
  data_in : Inport  Port=4  OutDataTypeStr=uint32
  valid_in : Inport  Port=5  OutDataTypeStr=boolean
  dataInCh1 : Inport  Port=6
  validInCh1 : Inport  Port=7
  access_per_burst : Inport  Port=8
  packetsPerBurst : Inport  Port=9
  " Zero" : Constant  Value=complex(0,0)  OutDataTypeStr=fixdt(1,16,15)  SampleTime=qam_params.symbolPeriod
  Async FIFO : Subsystem
  Code Unpacking : Subsystem
  Complex to Real-Imag2 : ComplexToRealImag
  Controller FSM1 : MATLAB Function  TreatAsAtomicUnit=on  SystemSampleTime=1/qam_params.symbolRate
  Delay : Delay  DelayLength=1  InitialCondition=0
  Enabled Subsystem : Subsystem  TreatAsAtomicUnit=on
  Input Mux : MultiPortSwitch  DataPortOrder=Zero-based contiguous  Inputs=2  zeroidx=on  SaturateOnIntegerOverflow=off  InputSameDT=off
  Logical Operator : Logic  Operator=NOT  AllPortsSameDT=off  OutDataTypeStr=boolean
  Packetization : Subsystem
  Pipeline{1..6,10..19} (16 alike) : Delay  DelayLength=1  InitialCondition=0
  Pipeline7 : Delay  InitialCondition=0
  Pipeline8 : Delay  InitialCondition=0
  Product1 : Product  OutDataTypeStr=fixdt(1,16,15)  RndMeth=Zero
  Pulse Shaping : Subsystem
  Rate Transition : RateTransition  InitialCondition=true  OutPortSampleTime=1/qam_params.symbolRate
  Repeat : dspsigops/Repeat  FactorSource=Dialog parameter  N=qam_params.Upsampling  Nmax=16  InputProcessing=Columns as channels (frame based)  RateOptions=Allow multirate processing  ic=0  mode=Unused parameter value
  Repeat1 : dspsigops/Repeat  FactorSource=Dialog parameter  N=qam_params.spreadingFactor  Nmax=16  InputProcessing=Columns as channels (frame based)  RateOptions=Allow multirate processing  ic=0  mode=Unused parameter value
  Repeat3 : dspsigops/Repeat  FactorSource=Dialog parameter  N=qam_params.spreadingFactor  Nmax=16  InputProcessing=Columns as channels (frame based)  RateOptions=Allow multirate processing  ic=0  mode=Unused parameter value
  Repeat4 : dspsigops/Repeat  FactorSource=Dialog parameter  N=qam_params.spreadingFactor  Nmax=16  InputProcessing=Columns as channels (frame based)  RateOptions=Allow multirate processing  ic=0  mode=Unused parameter value
  Subsystem2 : Subsystem
  Symbol Mapping : Subsystem
  Terminator{,1,3..4,6..7} (6 alike) : Terminator
  To Workspace : ToWorkspace  VariableName=yout26  SampleTime=-1
      settings: Save2DSignal=2-D array (concatenate along first dimension)
  To Workspace1 : ToWorkspace  VariableName=yout29  SampleTime=-1
      settings: Save2DSignal=2-D array (concatenate along first dimension)
  Data_Out : Outport  VectorParamsAs1DForOutWhenUnconnected=off
  Valid Out : Outport  Port=2  VectorParamsAs1DForOutWhenUnconnected=off
  axi_ready : Outport  Port=3
  wires:
  Pipeline10/1 -> Input Mux/1
  " Zero"/1 -> Input Mux/2
  Pulse Shaping/1(dataOut) -> Pipeline5/1
  Repeat/1 -> Pipeline6/1
  Pipeline6/1 -> Valid Out/1
  Symbol Mapping/1(Valid out) -> Pipeline10/1
  Pipeline2/1 -> Symbol Mapping/2(Integer In)
  Symbol Mapping/2(Symbol Out) -> Pipeline11/1
  Pipeline1/1 -> Symbol Mapping/1(Valid In)
  Pipeline11/1 -> Input Mux/3
  Code Unpacking/1(Out1) -> Product1/2, Pipeline18/1
  Repeat1/1 -> Product1/1
  Pipeline13/1 -> Packetization/1(Reset Preamble)
  Pipeline12/1 -> Packetization/2(Load Preamble)
  Pipeline4/1 -> Packetization/3(Data In)
  Pipeline15/1 -> Repeat/1
  Pipeline14/1 -> Pulse Shaping/1(dataIn)
  Controller FSM1/2(reset_preamble) -> Repeat4/1
  Controller FSM1/3(load_preamble) -> Repeat3/1
  Input Mux/1 -> Pipeline17/1
  Product1/1 -> Pipeline4/1
  Pipeline17/1 -> Repeat1/1
  codeSequence/1 -> Code Unpacking/1(code sequence)
  Packetization/2(Chip Out) -> Pipeline14/1
  Controller FSM1/1(valid) -> Terminator/1
  txEnable/1 -> Async FIFO/4(txEnable)
  Repeat3/1 -> Pipeline12/1
  Repeat4/1 -> Pipeline13/1
  Packetization/1(Valid out) -> Pipeline15/1
  Pipeline5/1 -> Complex to Real-Imag2/1, Data_Out/1
  Complex to Real-Imag2/1 -> Terminator3/1  "txShapedChips_Re"
  Complex to Real-Imag2/2 -> Terminator4/1  "txShapedChips_Im"
  Pipeline3/1 -> Pipeline1/1
  Pipeline16/1 -> Pipeline2/1
  Pipeline18/1 -> Packetization/4(Code In)
  txSrcSelect/1 -> Terminator1/1
  dataInCh1/1 -> Terminator7/1
  validInCh1/1 -> Terminator6/1
  Controller FSM1/4(load_data) -> Logical Operator/1, To Workspace/1, Pipeline7/1, Async FIFO/1(load_payload)
  Pipeline8/1 -> Pipeline16/1
  Pipeline7/1 -> Pipeline3/1
  Subsystem2/1(transmitNow) -> Controller FSM1/1(transmitNow)  "transmitNow"
  Pipeline19/1 -> Subsystem2/1(txEnable)
  data_in/1 -> Async FIFO/2(axi_data_in)
  valid_in/1 -> Async FIFO/3(axi_valid_in)
  Async FIFO/2(axi_ready_out) -> axi_ready/1
  Async FIFO/1(tx_enable) -> Pipeline19/1
  Async FIFO/3(payload_out) -> To Workspace1/1, Pipeline8/1
  access_per_burst/1 -> Async FIFO/5(access_per_burst)
  packetsPerBurst/1 -> Async FIFO/6(packets_per_burst), Rate Transition/1
  Rate Transition/1 -> Enabled Subsystem/1(In1)
  Enabled Subsystem/1(packetsPerBurst) -> Controller FSM1/2(packetsPerBurst)
  Delay/1 -> Enabled Subsystem/2(hold)
  Logical Operator/1 -> Delay/1

== system benchlink/HDL_64QAM/HDLRxIPCore/QAM Rx HDL/AGC Enable ==
  AGCEnable : Inport
  Constant19 : Constant  OutDataTypeStr=boolean  SampleTime=1/(qam_params.sampleRate)
  Constant20 : Constant  Value=0  OutDataTypeStr=boolean  SampleTime=1/(qam_params.sampleRate)
  Switch9 : Switch  Criteria=u2 ~= 0  SaturateOnIntegerOverflow=off  InputSameDT=off
  Unit Delay : UnitDelay  InitialCondition=int16(150)  SampleTime=-1  HasFrameUpgradeWarning=on
  Out : Outport  VectorParamsAs1DForOutWhenUnconnected=off
  wires:
  AGCEnable/1 -> Unit Delay/1
  Constant19/1 -> Switch9/1
  Unit Delay/1 -> Switch9/2
  Constant20/1 -> Switch9/3
  Switch9/1 -> Out/1

== system benchlink/HDL_64QAM/HDLRxIPCore/QAM Rx HDL/CFC Enable ==
  CFCEnable : Inport
  Constant19 : Constant  OutDataTypeStr=boolean  SampleTime=1/(qam_params.chipRate)
  Constant20 : Constant  Value=0  OutDataTypeStr=boolean  SampleTime=1/(qam_params.chipRate)
  Switch9 : Switch  Criteria=u2 ~= 0  SaturateOnIntegerOverflow=off  InputSameDT=off
  Unit Delay : UnitDelay  InitialCondition=int16(150)  SampleTime=-1  HasFrameUpgradeWarning=on
  Out : Outport  VectorParamsAs1DForOutWhenUnconnected=off
  wires:
  CFCEnable/1 -> Unit Delay/1
  Constant19/1 -> Switch9/1
  Unit Delay/1 -> Switch9/2
  Constant20/1 -> Switch9/3
  Switch9/1 -> Out/1

== system benchlink/HDL_64QAM/HDLRxIPCore/QAM Rx HDL/CFC Threshold ==
  CFCThreshold : Inport
  Bit Concat : hdlsllib/Logic and Bit Operations/Bit Concat  numInputs=7
  Bit Slice : hdlsllib/Logic and Bit Operations/Bit Slice  lidx=5  ridx=5
  Bit Slice1 : hdlsllib/Logic and Bit Operations/Bit Slice  lidx=4  ridx=4
  Bit Slice2 : hdlsllib/Logic and Bit Operations/Bit Slice  lidx=3  ridx=3
  Bit Slice3 : hdlsllib/Logic and Bit Operations/Bit Slice  lidx=2  ridx=2
  Bit Slice4 : hdlsllib/Logic and Bit Operations/Bit Slice  lidx=1  ridx=1
  Bit Slice5 : hdlsllib/Logic and Bit Operations/Bit Slice  lidx=0  ridx=0
  Bit Slice6 : hdlsllib/Logic and Bit Operations/Bit Slice  lidx=6  ridx=6
  Constant{6,8,10,12,14,16,18} (7 alike) : Constant  Value=0  OutDataTypeStr=boolean  SampleTime=1/(qam_params.chipRate)
  Constant{5,7,9,11,13,15,17} (7 alike) : Constant  OutDataTypeStr=boolean  SampleTime=1/(qam_params.chipRate)
  Scale : Gain  Gain=0.01  OutDataTypeStr=fixdt(0,16,15)  RndMeth=Zero
  Switch{1..7} (7 alike) : Switch  Criteria=u2 ~= 0  SaturateOnIntegerOverflow=off  InputSameDT=off
  Unit Delay : UnitDelay  InitialCondition=int16(150)  SampleTime=-1  HasFrameUpgradeWarning=on
  Threshold : Outport  VectorParamsAs1DForOutWhenUnconnected=off
  wires:
  Constant16/1 -> Switch6/3
  Bit Slice3/1 -> Switch5/2
  Constant17/1 -> Switch7/1
  Constant14/1 -> Switch5/3
  Bit Slice1/1 -> Switch3/2
  Constant13/1 -> Switch5/1
  Bit Slice4/1 -> Switch6/2
  Constant11/1 -> Switch4/1
  Bit Slice/1 -> Switch2/2
  Constant10/1 -> Switch3/3
  Bit Slice5/1 -> Switch7/2
  Bit Slice2/1 -> Switch4/2
  Constant18/1 -> Switch7/3
  Constant12/1 -> Switch4/3
  Constant6/1 -> Switch1/3
  Constant7/1 -> Switch2/1
  Constant15/1 -> Switch6/1
  Constant9/1 -> Switch3/1
  Bit Slice6/1 -> Switch1/2
  Constant5/1 -> Switch1/1
  Constant8/1 -> Switch2/3
  CFCThreshold/1 -> Unit Delay/1
  Bit Concat/1 -> Scale/1
  Unit Delay/1 -> Bit Slice6/1, Bit Slice/1, Bit Slice1/1, Bit Slice2/1, Bit Slice3/1, Bit Slice4/1, Bit Slice5/1
  Scale/1 -> Threshold/1
  Switch1/1 -> Bit Concat/1
  Switch7/1 -> Bit Concat/7
  Switch6/1 -> Bit Concat/6
  Switch5/1 -> Bit Concat/5
  Switch4/1 -> Bit Concat/4
  Switch3/1 -> Bit Concat/3
  Switch2/1 -> Bit Concat/2

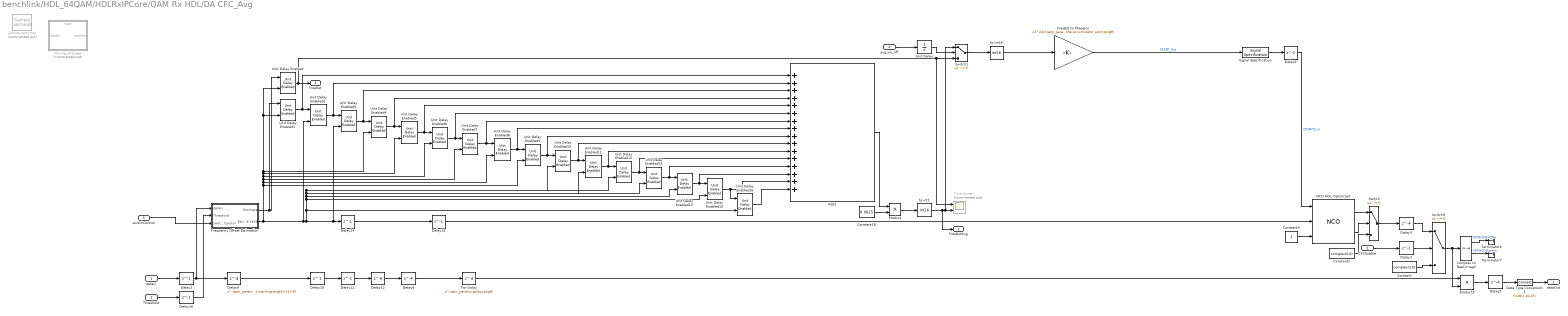
== system benchlink/HDL_64QAM/HDLRxIPCore/QAM Rx HDL/DA CFC_Avg ==
  dataIn : Inport  PortDimensions=1
  CFCEnable : Inport  Port=2  PortDimensions=1
  Threshold : Inport  Port=3
  avg_on_off : Inport  Port=4
  switchControl : Inport  Port=5
  Add1 : Sum  Inputs=++++++++++++++++  OutDataTypeStr=int32
  Complex to Real-Imag3 : ComplexToRealImag
  Constant : Constant  Value=complex(1,0)  OutDataTypeStr=fixdt(1,16,14)  SampleTime=1/(qam_params.chipRate)
  Constant18 : Constant  Value=0.0625  OutDataTypeStr=fixdt(1,16,14)  SampleTime=-1
  Constant2 : Constant  Value=complex(0,0)  OutDataTypeStr=fixdt(1,16,15)  SampleTime=1/(qam_params.chipRate)
  Constant4 : Constant  OutDataTypeStr=boolean  SampleTime=1/(qam_params.chipRate)
  Data Type Conversion1 : DataTypeConversion  OutDataTypeStr=fixdt(1,16,15)  SaturateOnIntegerOverflow=off  RndMeth=Floor
  Delay{1..2,6,10..11,14..16} (8 alike) : Delay  DelayLength=1  InitialCondition=0
  Delay12 : Delay  DelayLength=6  InitialCondition=0
  Delay3 : Delay  DelayLength=4  InitialCondition=0
  Delay5 : Delay  DelayLength=4  InitialCondition=0
  Delay8 : Delay  DelayLength=4  InitialCondition=0
  Delay9 : Delay  DelayLength=qam_params.trainingLength+21+35  InitialCondition=0
  For Golay : Delay  DelayLength=qam_params.golayLength  InitialCondition=0
  FreqEst to PhaseInc : Gain  Gain=-(2^24)/(qam_params.chipRate) %This converts the freq offset estimate to phase inc. 24 is the accumulator word length  OutDataTypeStr=fixdt(1,24,0)
  Frequency Offset Estimation : Subsystem
  Moving_Average : Subsystem  Commented=on
  NCO HDL Optimized : dsphdlsigops2/NCO  PhaseIncrementSource=Input port  PhaseIncrement=100  PhaseOffsetSource=Property  PhaseOffset=0  DitherSource=Property  NumDitherBits=4  SamplesPerFrame=1  LUTCompress=on  ResetAction=on  Waveform=Complex exponential  PhasePort=off  SimulateUsing=Code generation  AccumulatorWL=24  PhaseQuantization=on  NumQuantizerAccumulatorBits=17  OutputDataType=Binary point scaling  OutputWL=16  OutputFL=15
  Product : Product
  Product3 : Product  RndMeth=Zero  SaturateOnIntegerOverflow=on
  Sample and Hold : dspsigops/Sample and Hold  Commented=on  trig=Rising edge  initCond=0  latchinput=off
  Signal Specification : SignalSpecification  OutDataTypeStr=fixdt(1,24,0)  Dimensions=1
  Switch : Switch  Criteria=u2 ~= 0  SaturateOnIntegerOverflow=off  InputSameDT=off
  Switch1 : Switch  Criteria=u2 ~= 0  SaturateOnIntegerOverflow=off  InputSameDT=off
  Switch9 : Switch  Criteria=u2 ~= 0  SaturateOnIntegerOverflow=off  InputSameDT=off
  Terminator6 : Terminator
  Terminator7 : Terminator
  Time Scope : Scope  Commented=on  NumInputPorts=2
  Unit Delay : UnitDelay  InitialCondition=int16(150)  SampleTime=-1  HasFrameUpgradeWarning=on
  Unit Delay Enabled{,1..16} (17 alike) : simulink_need_slupdate/Unit Delay Enabled  vinit=0.0  tsamp=-1
  to int1 : DataTypeConversion  OutDataTypeStr=int16  RndMeth=Floor
  to int16 : DataTypeConversion  OutDataTypeStr=int16  RndMeth=Floor
  dataOut : Outport  VectorParamsAs1DForOutWhenUnconnected=off
  FreqEst : Outport  Port=2  VectorParamsAs1DForOutWhenUnconnected=off
  FreqEstAvg : Outport  Port=3  VectorParamsAs1DForOutWhenUnconnected=off
  wires:
  Data Type Conversion1/1 -> dataOut/1
  Threshold/1 -> Delay16/1
  Delay5/1 -> Data Type Conversion1/1
  Frequency Offset Estimation/1(Estimate) -> Unit Delay Enabled/1, Unit Delay Enabled1/1
  dataIn/1 -> Delay2/1
  Product3/1 -> Delay5/1
  CFCEnable/1 -> Delay1/1
  Switch/1 -> Delay3/1
  Constant2/1 -> Switch/3
  NCO HDL Optimized/1 -> Switch/1
  Signal Specification/1 -> Delay6/1
  FreqEst to PhaseInc/1 -> Signal Specification/1  "CFCFP_Out"
  Complex to Real-Imag3/2 -> Terminator7/1  "CFCNCOOut_Im"
  Unit Delay Enabled1/1 -> Add1/1, Unit Delay Enabled2/1
  Delay10/1 -> Delay11/1
  Complex to Real-Imag3/1 -> Terminator6/1  "CFCNCOOut_Re"
  For Golay/1 -> Product3/1
  Delay1/1 -> Switch9/2
  to int16/1 -> FreqEst to PhaseInc/1
  Delay12/1 -> Delay8/1
  Unit Delay/1 -> Switch1/2
  Delay2/1 -> Delay9/1, Frequency Offset Estimation/1(dataIn)
  Constant18/1 -> Product/2
  Unit Delay Enabled16/1 -> Add1/16
  Delay15/1 -> NCO HDL Optimized/2
  Switch9/1 -> Complex to Real-Imag3/1, Product3/2
  Delay16/1 -> Frequency Offset Estimation/2(Threshold)
  Switch1/1 -> to int16/1
  NCO HDL Optimized/2 -> Switch/2
  avg_on_off/1 -> Unit Delay/1
  Product/1 -> to int1/1
  Delay11/1 -> Delay12/1
  Constant4/1 -> NCO HDL Optimized/3
  Delay3/1 -> Switch9/1
  Add1/1 -> Product/1
  Delay9/1 -> Delay10/1
  Delay14/1 -> Delay15/1
  Delay8/1 -> For Golay/1
  Delay6/1 -> NCO HDL Optimized/1  "CFCNCO_In"
  Constant/1 -> Switch9/3
  to int1/1 -> Switch1/1, Time Scope/2, FreqEstAvg/1
  Unit Delay Enabled10/1 -> Unit Delay Enabled11/1, Add1/10
  Unit Delay Enabled2/1 -> Add1/2, Unit Delay Enabled3/1
  Unit Delay Enabled3/1 -> Add1/3, Unit Delay Enabled4/1
  Frequency Offset Estimation/2(Estimate Valid) -> Delay14/1, Unit Delay Enabled3/2, Unit Delay Enabled12/2, Unit Delay Enabled10/2, Unit Delay Enabled11/2, Unit Delay Enabled13/2, Unit Delay Enabled14/2, Unit Delay Enabled15/2, Unit Delay Enabled16/2, Unit Delay Enabled2/2, Unit Delay Enabled/2, Unit Delay Enabled1/2, Unit Delay Enabled4/2, Unit Delay Enabled5/2, Unit Delay Enabled6/2, Unit Delay Enabled7/2, Unit Delay Enabled8/2, Unit Delay Enabled9/2
  Unit Delay Enabled4/1 -> Add1/4, Unit Delay Enabled5/1
  Unit Delay Enabled5/1 -> Unit Delay Enabled6/1, Add1/5
  Unit Delay Enabled6/1 -> Add1/6, Unit Delay Enabled7/1
  Unit Delay Enabled7/1 -> Unit Delay Enabled8/1, Add1/7
  Unit Delay Enabled14/1 -> Unit Delay Enabled15/1, Add1/14
  Unit Delay Enabled15/1 -> Unit Delay Enabled16/1, Add1/15
  Unit Delay Enabled9/1 -> Unit Delay Enabled10/1, Add1/9
  Unit Delay Enabled13/1 -> Unit Delay Enabled14/1, Add1/13
  Unit Delay Enabled12/1 -> Unit Delay Enabled13/1, Add1/12
  Unit Delay Enabled11/1 -> Unit Delay Enabled12/1, Add1/11
  Unit Delay Enabled8/1 -> Unit Delay Enabled9/1, Add1/8
  Unit Delay Enabled/1 -> Switch1/3, Time Scope/1, FreqEst/1
  switchControl/1 -> Frequency Offset Estimation/3(switchControl)

== system benchlink/HDL_64QAM/HDLRxIPCore/QAM Rx HDL/EB Downsampler by 6 ==
  dataIn : Inport  PortDimensions=1
  Delay{1..2,6,11..12,33..37} (10 alike) : Delay  DelayLength=1  InitialCondition=0
  Delay4 : Delay  DelayLength=floor(M/2)+1  InitialCondition=0
  Delay5 : Delay  DelayLength=4  InitialCondition=0
  Downsample : DownSample  N=6  RateOptions=Allow multirate processing
  Maximum : dspstat3/Maximum  operation=maximum  fcn=Index  indexBase=One  operateOver=Each column  Dimension=1  InputProcessing=Columns as channels (frame based)  reset=None  roiEnable=off  roiType=Rectangles  roiPortion=Entire ROI  roiOutput=Individual statistics for each ROI  roiFlag=off  roundingMode=Floor  overflowMode=off  accumDataTypeStr=Inherit: Same as product output  accumLastDataTypeStr=Inherit: Same as product output
  Modulus : Subsystem
  Moving_Average : Subsystem
  Selector : Selector  InputPortWidth=6  IndexOptions=Index vector (port)  Indices=[1 3]  OutputSizes=1
  Vector Concatenate : Concatenate  NumInputs=6
  dataOut : Outport  VectorParamsAs1DForOutWhenUnconnected=off
  wires:
  dataIn/1 -> Delay2/1
  Delay11/1 -> dataOut/1
  Delay2/1 -> Delay33/1, Vector Concatenate/1
  Delay33/1 -> Delay34/1, Vector Concatenate/2
  Delay34/1 -> Vector Concatenate/3, Delay35/1
  Delay35/1 -> Vector Concatenate/4, Delay36/1
  Delay36/1 -> Vector Concatenate/5, Delay37/1
  Delay37/1 -> Vector Concatenate/6
  Vector Concatenate/1 -> Downsample/1
  Downsample/1 -> Delay1/1
  Modulus/1(dataOut) -> Moving_Average/1(dataIn)
  Delay1/1 -> Delay5/1, Modulus/1(dataIn)
  Delay6/1 -> Maximum/1
  Moving_Average/1(dataOut) -> Delay6/1
  Maximum/1 -> Selector/2  "DS6PortSel_Out"
  Selector/1 -> Delay11/1
  Delay4/1 -> Delay12/1
  Delay5/1 -> Delay4/1
  Delay12/1 -> Selector/1
